simulink model "TParkInv"  (R2020b)
settings: Solver=VariableStepAuto  StartTime=0.0  StopTime=10.0  RelTol=1e-3
values from neighbouring files (symbols this model uses):
  beq = bm+(blnom/(r^2))    (= 1.5e-05)    [valores.m]
  Jeq = (Jm+Jl/r^2)    (= 5.65099476805e-06)    [Valores_de_Parametros.m]    (also in valores.m)
  lambda_m = 0.01546    [Valores_de_Parametros.m]    (also in valores.m)
  Ld = 6.6    [Valores_de_Parametros.m]    (also in valores.m = 0.0066)
  Lls = 0.8    [Valores_de_Parametros.m]    (also in valores.m = 0.0008)
  Lq = 5.8    [Valores_de_Parametros.m]    (also in valores.m = 0.0058)
  Pp = 3    [Valores_de_Parametros.m]    (also in valores.m)
  r = 314.3008    [Valores_de_Parametros.m]    (also in valores.m)
  Rs = 1.02    [Valores_de_Parametros.m]    (also in valores.m)
settings Model: Creator=Matias  LastModifiedBy=Matias

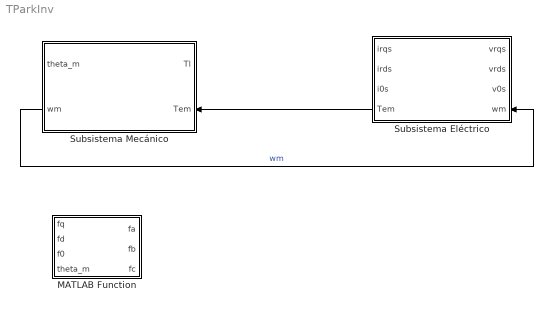
== system TParkInv ==
  MATLAB Function : MATLAB Function  TreatAsAtomicUnit=on
  Subsistema Eléctrico : Subsystem
  Subsistema Mecánico : Subsystem
  wires:
  Subsistema Mecánico/2(wm) -> Subsistema Eléctrico/4(wm)  "wm"
  Subsistema Eléctrico/4(Tem) -> Subsistema Mecánico/2(Tem)

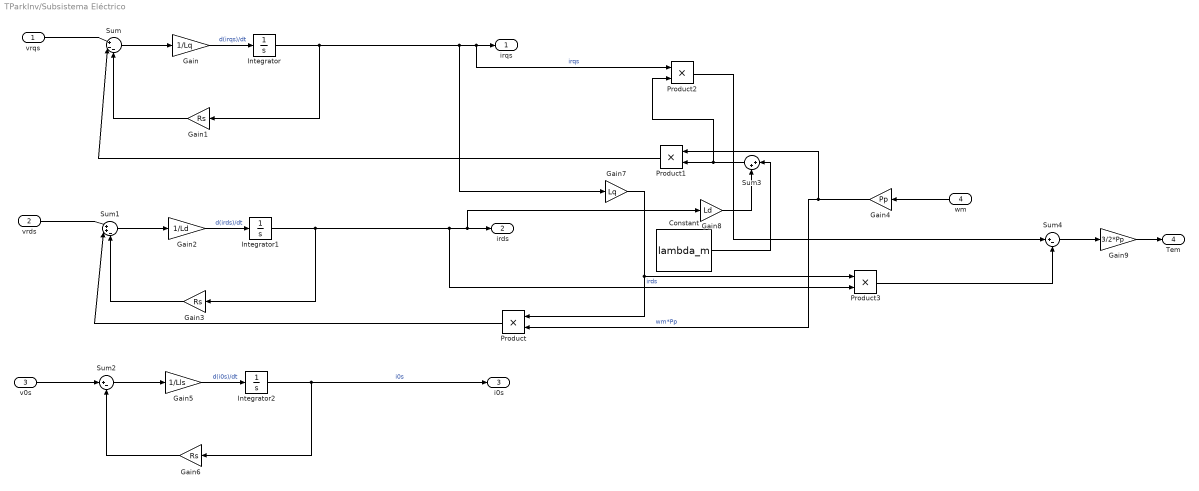
== system TParkInv/Subsistema Eléctrico ==
  vrqs : Inport
  vrds : Inport  Port=2
  v0s : Inport  Port=3
  wm : Inport  Port=4
  Constant : Constant  Value=lambda_m
  Gain : Gain  Gain=1/Lq
  Gain1 : Gain  Gain=Rs
  Gain2 : Gain  Gain=1/Ld
  Gain3 : Gain  Gain=Rs
  Gain4 : Gain  Gain=Pp
  Gain5 : Gain  Gain=1/Lls
  Gain6 : Gain  Gain=Rs
  Gain7 : Gain  Gain=Lq
  Gain8 : Gain  Gain=Ld
  Gain9 : Gain  Gain=3/2*Pp
  Integrator : Integrator
  Integrator1 : Integrator
  Integrator2 : Integrator
  Product{,1..3} (4 alike) : Product
  Sum : Sum  Inputs=|+--
  Sum1 : Sum  Inputs=|++-
  Sum2 : Sum  Inputs=|+-
  Sum3 : Sum  Inputs=|++
  Sum4 : Sum  Inputs=|+-
  irqs : Outport
  irds : Outport  Port=2
  i0s : Outport  Port=3
  Tem : Outport  Port=4
  wires:
  Sum3/1 -> Product2/2, Product1/2
  Integrator1/1 -> Gain3/1, Product3/2, Gain8/1, irds/1  "irds"
  Sum1/1 -> Gain2/1
  Gain8/1 -> Sum3/2
  Gain2/1 -> Integrator1/1  "d(irds)/dt"
  Product2/1 -> Sum4/1
  Constant/1 -> Sum3/1
  Gain3/1 -> Sum1/3
  Sum4/1 -> Gain9/1
  Product3/1 -> Sum4/2
  vrqs/1 -> Sum/1
  wm/1 -> Gain4/1
  vrds/1 -> Sum1/1
  Product/1 -> Sum1/2
  Product1/1 -> Sum/2
  v0s/1 -> Sum2/1
  Gain5/1 -> Integrator2/1  "d(i0s)/dt"
  Sum2/1 -> Gain5/1
  Integrator2/1 -> Gain6/1, i0s/1  "i0s"
  Gain4/1 -> Product1/1, Product/2  "wm*Pp"
  Sum/1 -> Gain/1
  Gain1/1 -> Sum/3
  Gain7/1 -> Product/1, Product3/1
  Integrator/1 -> Gain1/1, Gain7/1, Product2/1, irqs/1  "irqs"
  Gain/1 -> Integrator/1  "d(irqs)/dt"
  Gain9/1 -> Tem/1
  Gain6/1 -> Sum2/2

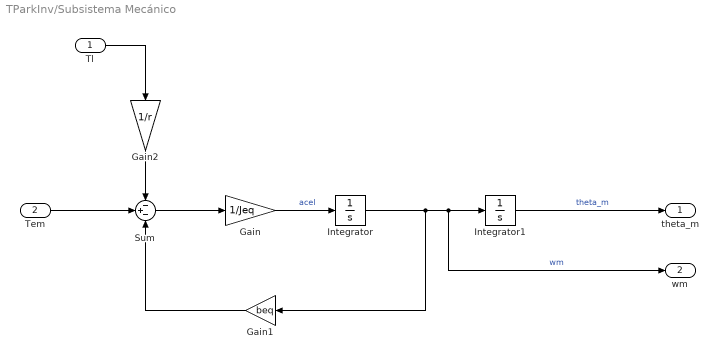
== system TParkInv/Subsistema Mecánico ==
  Tl : Inport
  Tem : Inport  Port=2
  Gain : Gain  Gain=1/Jeq
  Gain1 : Gain  Gain=beq
  Gain2 : Gain  Gain=1/r
  Integrator : Integrator
  Integrator1 : Integrator
  Sum : Sum  Inputs=-+-
  theta_m : Outport
  wm : Outport  Port=2
  wires:
  Sum/1 -> Gain/1
  Tl/1 -> Gain2/1
  Gain1/1 -> Sum/3
  Integrator/1 -> Gain1/1, wm/1, Integrator1/1  "wm"
  Gain2/1 -> Sum/1
  Gain/1 -> Integrator/1  "acel"
  Integrator1/1 -> theta_m/1  "theta_m"
  Tem/1 -> Sum/2

== matlab function TParkInv/MATLAB Function ==
  data: fq input; fa output; fd input; f0 input; theta_m input; fb output; fc output
function [fa,fb,fc] = fcn(fq,fd,f0,theta_m)
fa=fq*cos(theta_m)+fd*sin(theta_m)+f0;
fb=fq*cos(theta_m-(2*pi/(3)))+fd*sin(theta_m-(2*pi/(3)))+f0;
fc=fq*cos(theta_m+(2*pi/(3)))+fd*sin(theta_m+(2*pi/(3)))+f0;
